simulink model "predictive_controller"  (R2019b)
settings: Solver=VariableStepAuto  StartTime=0.0  StopTime=10.0  RelTol=1e-3
settings Model: Creator=PC  LastModifiedBy=PC

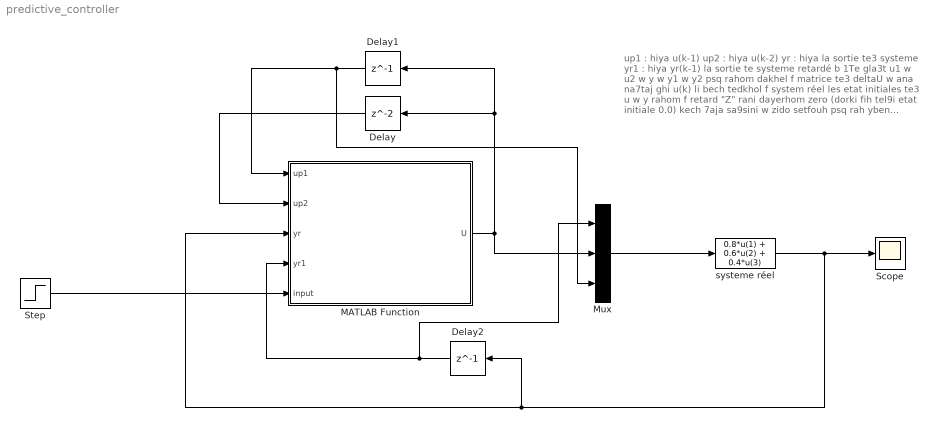
== system predictive_controller ==
  note: up1 : hiya u(k-1)
      | up2 : hiya u(k-2)
      | yr : hiya la sortie te3 systeme
      | yr1 : hiya yr(k-1) la sortie te systeme retardé b 1Te
      | gla3t u1 w u2 w y w y1 w y2 psq rahom dakhel f matrice te3
      | deltaU w ana na7taj ghi u(k) li bech tedkhol f system réel
      |
      | les etat initiales te3 u w y rahom f retard "Z" rani dayerhom
      | zero (dorki fih tel9i etat initiale 0.0)
      | kech 7aja sa9sini w zido setfouh psq rah yben mkharbech
      | bon courage
  Delay : Delay
  Delay1 : Delay  DelayLength=1
  Delay2 : Delay  DelayLength=1
  MATLAB Function : MATLAB Function  TreatAsAtomicUnit=on
  Mux : Mux  Inputs=3
  Scope : Scope
  Step : Step  SampleTime=0
  "systeme réel " : Fcn  Expr=0.8*u(1) + 0.6*u(2) + 0.4*u(3)
  wires:
  Delay/1 -> MATLAB Function/2(up2)
  Delay1/1 -> Mux/3, MATLAB Function/1(up1)
  Step/1 -> MATLAB Function/5(input)
  "systeme réel "/1 -> Delay2/1, MATLAB Function/3(yr), Scope/1
  Delay2/1 -> Mux/1, MATLAB Function/4(yr1)
  Mux/1 -> "systeme réel "/1
  MATLAB Function/1(U) -> Delay1/1, Delay/1, Mux/2

== matlab function predictive_controller/MATLAB Function ==
  data: up1 input; U output; up2 input; yr input; yr1 input; input input
function U = fcn(up1,up2,yr,yr1,input)
w = input;
G = [0.4 0 0; 1.32 0.4 0; 2.056 1.32 0.4];
lambda = 0.8;
F = [0.6*(up1-up2)+1.8*yr-0.8*yr1;1.08*(up1-up2)+2.44*yr-1.44*yr1;1.464*(up1-up2)+2.952*yr-1.952*yr1];
deltaU = -(inv(G'*G + lambda*eye(3))*G')*(F-[w;w;w]);
U = deltaU(1)+up1;
